simulink model "atrias_HW_boom_nmSt_kinSw_v3"  (R2015a)
settings: Solver=ode4  StartTime=0.0  StopTime=inf  FixedStep=sample_time  RelTol=1e-3
values from neighbouring files (symbols this model uses):
  control_start_time = 15    [setParams.m]
  flag_CtrlMode = 0    [setParams.m]
  kinSw_alpha_start = 130*pi/180    (= 2.26892802759)    [setParams.m]
  kinSw_alpha_tgt = 70*pi/180    (= 1.2217304764)    [setParams.m]
  kinSw_t_start = 0.5    [setParams.m]
  poser_LLegAlp = (initial_l_leg_angle -pi/2)*180/pi    (= 105)    [setParams.m]
  poser_LLegLen = initial_l_leg_length    (= 0.8)    [setParams.m]
  poser_RLegAlp = (initial_r_leg_angle -pi/2)*180/pi    (= 75)    [setParams.m]
  poser_RLegLen = initial_r_leg_length    (= 0.8)    [setParams.m]
  tune_kinSw_alpha_start = kinSw_alpha_start*180/pi    (= 130)    [setParams.m]
  tune_kinSw_alpha_tgt = kinSw_alpha_tgt*180/pi    (= 70)    [setParams.m]
  tune_kinSw_len_min = kinSw_len_min    (= 0.6)    [setParams.m]
  tune_kinSw_len_tgt = kinSw_len_tgt    (= 0.9)    [setParams.m]
  tune_M1_G = 9.5    [setParams.m]
  tune_M3_0 = CtrlPar_theta0*180/pi    [setParams.m]
  tune_M3_D = St_GainDTh_HFL*5    [setParams.m]
  tune_M3_P = St_GainTh_HFL*5    [setParams.m]
  tune_M4_G = 1    [setParams.m]
undefined symbols (not defined in the file or in its folder): A1_notch_f1, A2_notch_f1, A_kalman_fourbar_gear, A_lpf_dtau, B1_lpf_dtau, B1_notch_f1, B2_lpf_dtau, B2_notch_f1, B_kalman_fourbar_gear, boom_mount_angle, boom_mount_to_center_diagonal, c_jointstop, C_kalman_fourbar_gear, contactThr, d_vertical_com, delta_phi_max, delta_phi_max_buffer, delta_phi_max_dropoff, delta_phi_min, Discrete, FmaxBFSH, FmaxGLU, FmaxHAM, FmaxHFL, FmaxRF, FmaxVAS, FPCtrlPar, g, gain_nodes_sea_torque, HIP_MTR_MAX_CONT_TORQUE, initial_dx_estimate, j_motor, k_leg_spring, K_notch_f1, k_sea, kalman_load_to_deflect_transmission, kd_lateral, kd_motor, kd_shin_max, kd_shin_min, kd_splay_max, kd_splay_min, kd_thigh_max, kd_thigh_min, kp_lateral, kp_motor, kp_sea_torque, kp_shin_max, kp_shin_min, kp_splay_max, kp_splay_min, kp_thigh_max, kp_thigh_min, l_boom, l_seg, l_v, lateral_motor_efficiency, lateral_offset, lateral_target_angle_right, lateral_transition_force ... (+123)
libraries: simulink_extras x28, simulink x11, ctrlSharedLib x4
(part 3 of 8)

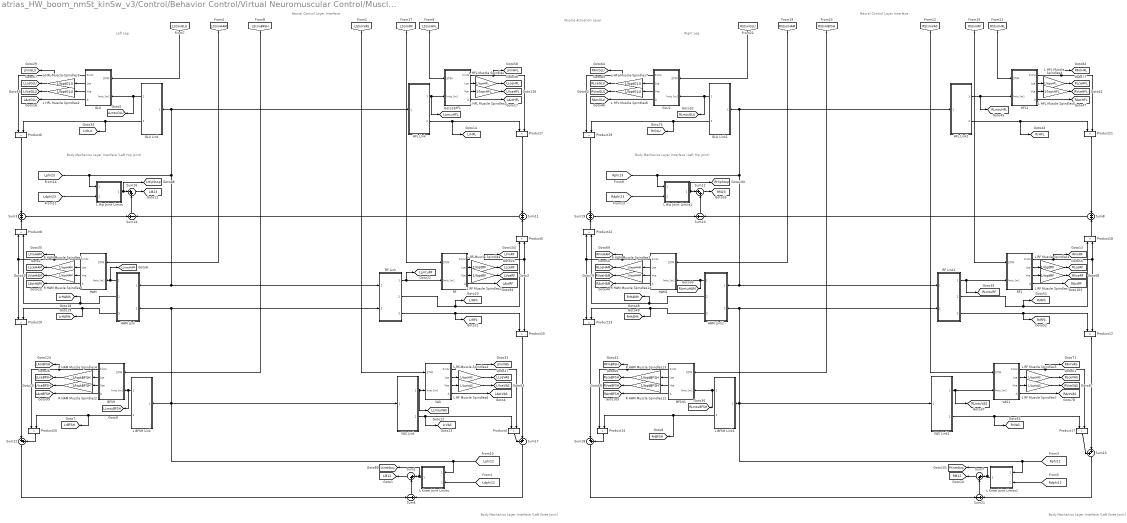
== system atrias_HW_boom_nmSt_kinSw_v3/Control/Behavior Control/Virtual Neuromuscular Control/Muscle Layer ==
  note: Left Leg
  note: Neural Control Layer Interface
  note: Muscle Actuation Layer
  note: Body Mechanics Layer
      | Interface (Left Hip Joint)
  note: Body Mechanics Layer
      | Interface (Left Knee Joint)
  note: Right Leg
  note: Neural Control Layer Interface
  note: Body Mechanics Layer
      | Interface (Left Hip Joint)
  note: Body Mechanics Layer
      | Interface (Left Knee Joint)
  BFSH : Subsystem
  BFSH1 : Subsystem
  GLU : Subsystem
  GLU Link : Subsystem
  GLU Link1 : Subsystem
  GLU1 : Subsystem
  HAM : Subsystem
  HAM Link : Subsystem
  HAM Link1 : Subsystem
  HAM1 : Subsystem
  HFL : Subsystem
  HFL Link : Subsystem
  HFL Link1 : Subsystem
  HFL1 : Subsystem
  L BFSH Link : Subsystem
  L BFSH Link1 : Subsystem
  L HFL Muscle Spindles{,1,4..5} (4 alike) : Gain  Gain=1/loptHFL
  L HFL Muscle Spindles{2..3,6..7} (4 alike) : Gain  Gain=1/loptGLU
  L Hip Joint Limits : Subsystem
  L Hip Joint Limits1 : Subsystem
  L Knee Joint Limits : Subsystem
  L Knee Joint Limits1 : Subsystem
  L RF Muscle Spindles{,1..3} (4 alike) : Gain  Gain=1/loptRF
  L RF Muscle Spindles{4..7} (4 alike) : Gain  Gain=1/loptVAS
  Product{4..9,12,14..15,17..23} (16 alike) : Product  RndMeth=Zero
  R HAM Muscle Spindles{1,3,6,14} (4 alike) : Gain  Gain=1/loptHAM
  R HAM Muscle Spindles{2,4,12..13} (4 alike) : Gain  Gain=1/loptBFSH
  RF : Subsystem
  RF Link : Subsystem
  RF Link1 : Subsystem
  RF1 : Subsystem
  Sum{1,7,12,16,18,22} (6 alike) : Sum  Inputs=|++
  Sum10 : Sum  Inputs=+-
  Sum{3,8,11,19} (4 alike) : Sum
  Sum13 : Sum  Inputs=++|
  Sum14 : Sum  Inputs=+-
  Sum17 : Sum  Inputs=++|
  Sum21 : Sum  Inputs=-+
  Sum5 : Sum  Inputs=-+
  VAS : Subsystem
  VAS Link : Subsystem
  VAS Link1 : Subsystem
  VAS1 : Subsystem
  tag scope: LActBFSH=global, LActGLU=global, LActHAM=global, LActHFL=global, LActRF=global, LActVAS=global, LFmBFSH=global, LFmGLU=global, LFmHAM=global, LFmHFL=global, LFmRF=global, LFmVAS=global, LHipStop=global, LKneeStop=global, LLceBFSH=global, LLceGLU=global, LLceHAM=global, LLceHFL=global, LLceRF=global, LLceVAS=global, LLmtuBFSH=global, LLmtuGLU=global, LLmtuHAM=global, LLmtuHFL=global, LLmtuRF=global, LLmtuVAS=global, LM12=global, LM23=global, LVceBFSH=global, LVceGLU=global, LVceHAM=global, LVceHFL=global, LVceRF=global, LVceVAS=global, LrBFSH=global, LrGLU=global, LrHAMh=global, LrHAMk=global, LrHFL=global, LrRFh=global, LrRFk=global, LrVAS=global, RActBFSH=global, RActGLU=global, RActHAM=global, RActHFL=global, RActRF=global, RActVAS=global, RFmBFSH=global, RFmGLU=global, RFmHAM=global, RFmHFL=global, RFmRF=global, RFmVAS=global, RHipStop=global, RKneeStop=global, RLceBFSH=global, RLceGLU=global, RLceHAM=global, RLceHFL=global, RLceRF=global, RLceVAS=global, RLmtuBFSH=global, RLmtuGLU=global, RLmtuHAM=global, RLmtuHFL=global, RLmtuRF=global, RLmtuVAS=global, RM12=global, RM23=global, RVceBFSH=global, RVceGLU=global, RVceHAM=global, RVceHFL=global, RVceRF=global, RVceVAS=global, RrBFSH=global, RrGLU=global, RrHAMh=global, RrHAMk=global, RrHFL=global, RrRFh=global, RrRFk=global, RrVAS=global
  wires:
  [Lphi12] -> L Knee Joint Limits/1(phi [rad]1), VAS Link/1(phi23 [rad]), RF Link/2(phi23 [rad]), HAM Link/2(phi23 [rad]), L BFSH Link/1(phi23 [rad])
  [LStimHAM] -> HAM/1(STIM)
  HAM/1(Fmtc) -> Product9/1, Product8/1, [LFmHAM]
  HAM/2(Lce) -> R HAM Muscle Spindles1/1
  HFL/1(Fmtc) -> Product7/2, [LFmHFL]
  HFL/2(Lce) -> L HFL Muscle Spindles/1
  [LStimHFL] -> HFL/1(STIM)
  GLU/1(Fmtc) -> Product6/1, [LFmGLU]
  [LStimGLU] -> GLU/1(STIM)
  Sum16/1 -> [LM23]
  [Ldphi12] -> L Knee Joint Limits/2(dphi [rad/s]1)
  VAS Link/1(lmtu [m]) -> VAS/2(lmtc [m]), [LLmtuVAS]
  HAM Link/1(lmtu [m]) -> HAM/2(lmtc [m]), [LLmtuHAM]
  HAM Link/2(lever34 [m]) -> Product8/2, [LrHAMh]
  HAM Link/3(lever23 [m]) -> Product9/2, [LrHAMk]
  Sum3/1 -> Sum14/1
  [Lphi23] -> L Hip Joint Limits/1(phi [rad]1), HFL Link/1(phi34 [rad]), GLU Link/1(phi34 [rad]), RF Link/1(phi34 [rad]), HAM Link/1(phi34 [rad])
  VAS/4(A) -> [LActVAS]
  VAS/1(Fmtc) -> Product4/2, [LFmVAS]
  Sum1/1 -> [LM12]
  L Knee Joint Limits/1(M_stop [Nm]1) -> Sum1/1, [LKneeStop]
  Sum5/1 -> Sum1/2
  VAS Link/2(lever [m]) -> [LrVAS], Product4/1
  Sum22/1 -> Sum5/1
  HAM/4(A) -> [LActHAM]
  Product8/1 -> Sum3/2
  Product6/1 -> Sum3/1
  GLU Link/1(lmtu [m]) -> GLU/2(lmtc [m]), [LLmtuGLU]
  GLU Link/2(lever [m]) -> Product6/2, [LrGLU]
  GLU/4(A) -> [LActGLU]
  [Ldphi23] -> L Hip Joint Limits/2(dphi [rad/s]1)
  L Hip Joint Limits/1(M_stop [Nm]1) -> [LHipStop], Sum16/1
  Sum14/1 -> Sum16/2
  HFL Link/1(lmtu [m]) -> HFL/2(lmtc [m]), [LLmtuHFL]
  HFL/4(A) -> [LActHFL]
  HFL Link/2(lever [m]) -> Product7/1, [LrHFL]
  [LStimVAS] -> VAS/1(STIM)
  GLU/2(Lce) -> L HFL Muscle Spindles3/1
  GLU/3(Vce) -> L HFL Muscle Spindles2/1
  HAM/3(Vce) -> R HAM Muscle Spindles6/1
  VAS/3(Vce) -> L RF Muscle Spindles6/1
  VAS/2(Lce) -> L RF Muscle Spindles4/1
  HFL/3(Vce) -> L HFL Muscle Spindles1/1
  RF/4(A) -> [LActRF]
  RF/3(Vce) -> L RF Muscle Spindles2/1
  RF/2(Lce) -> L RF Muscle Spindles/1
  RF Link/1(lmtu [m]) -> [LLmtuRF], RF/2(lmtc [m])
  RF Link/2(lever34 [m]) -> Product5/1, [LrRFh]
  RF Link/3(lever23 [m]) -> Product15/1, [LrRFk]
  [LStimRF] -> RF/1(STIM)
  Product7/1 -> Sum11/1
  Product5/1 -> Sum11/2
  Product15/1 -> Sum17/2
  Sum17/1 -> Sum5/2
  Product4/1 -> Sum17/1
  [LStimBFSH] -> BFSH/1(STIM)
  L BFSH Link/1(lmtu [m]) -> BFSH/2(lmtc [m]), [LLmtuBFSH]
  L BFSH Link/2(lever [m]) -> [LrBFSH], Product20/2
  BFSH/4(A) -> [LActBFSH]
  BFSH/2(Lce) -> R HAM Muscle Spindles4/1
  BFSH/3(Vce) -> R HAM Muscle Spindles2/1
  Product20/1 -> Sum22/2
  Product9/1 -> Sum22/1
  L HFL Muscle Spindles1/1 -> [LVceHFL]
  L HFL Muscle Spindles2/1 -> [LVceGLU]
  L HFL Muscle Spindles3/1 -> [LLceGLU]
  L RF Muscle Spindles6/1 -> [LVceVAS]
  RF/1(Fmtc) -> Product5/2, Product15/2, [LFmRF]
  BFSH/1(Fmtc) -> Product20/1, [LFmBFSH]
  L HFL Muscle Spindles/1 -> [LLceHFL]
  R HAM Muscle Spindles1/1 -> [LLceHAM]
  R HAM Muscle Spindles6/1 -> [LVceHAM]
  L RF Muscle Spindles/1 -> [LLceRF]
  L RF Muscle Spindles2/1 -> [LVceRF]
  R HAM Muscle Spindles4/1 -> [LLceBFSH]
  R HAM Muscle Spindles2/1 -> [LVceBFSH]
  L RF Muscle Spindles4/1 -> [LLceVAS]
  [Rphi12] -> L Knee Joint Limits1/1(phi [rad]1), VAS Link1/1(phi23 [rad]), HAM Link1/2(phi23 [rad]), RF Link1/2(phi23 [rad]), L BFSH Link1/1(phi23 [rad])
  [RStimHAM] -> HAM1/1(STIM)
  HAM1/1(Fmtc) -> Product23/1, Product22/1, [RFmHAM]
  HAM1/2(Lce) -> R HAM Muscle Spindles3/1
  HFL1/1(Fmtc) -> Product21/2, [RFmHFL]
  HFL1/2(Lce) -> L HFL Muscle Spindles4/1
  [RStimHFL] -> HFL1/1(STIM)
  GLU1/1(Fmtc) -> Product19/1, [RFmGLU]
  [RStimGLU] -> GLU1/1(STIM)
  Sum12/1 -> [RM23]
  [Rdphi12] -> L Knee Joint Limits1/2(dphi [rad/s]1)
  VAS Link1/1(lmtu [m]) -> VAS1/2(lmtc [m]), [RLmtuVAS]
  HAM Link1/1(lmtu [m]) -> HAM1/2(lmtc [m]), [RLmtuHAM]
  HAM Link1/2(lever34 [m]) -> Product22/2, [RrHAMh]
  HAM Link1/3(lever23 [m]) -> Product23/2, [RrHAMk]
  Sum19/1 -> Sum10/1
  [Rphi23] -> L Hip Joint Limits1/1(phi [rad]1), HFL Link1/1(phi34 [rad]), GLU Link1/1(phi34 [rad]), RF Link1/1(phi34 [rad]), HAM Link1/1(phi34 [rad])
  VAS1/4(A) -> [RActVAS]
  VAS1/1(Fmtc) -> Product17/2, [RFmVAS]
  Sum7/1 -> [RM12]
  L Knee Joint Limits1/1(M_stop [Nm]1) -> Sum7/1, [RKneeStop]
  Sum21/1 -> Sum7/2
  VAS Link1/2(lever [m]) -> [RrVAS], Product17/1
  Sum18/1 -> Sum21/1
  HAM1/4(A) -> [RActHAM]
  Product22/1 -> Sum19/2
  Product19/1 -> Sum19/1
  GLU Link1/1(lmtu [m]) -> GLU1/2(lmtc [m]), [RLmtuGLU]
  GLU Link1/2(lever [m]) -> Product19/2, [RrGLU]
  GLU1/4(A) -> [RActGLU]
  [Rdphi23] -> L Hip Joint Limits1/2(dphi [rad/s]1)
  L Hip Joint Limits1/1(M_stop [Nm]1) -> [RHipStop], Sum12/1
  Sum10/1 -> Sum12/2
  HFL Link1/1(lmtu [m]) -> [RLmtuHFL], HFL1/2(lmtc [m])
  HFL1/4(A) -> [RActHFL]
  HFL Link1/2(lever [m]) -> Product21/1, [RrHFL]
  [RStimVAS] -> VAS1/1(STIM)
  GLU1/2(Lce) -> L HFL Muscle Spindles7/1
  GLU1/3(Vce) -> L HFL Muscle Spindles6/1
  HAM1/3(Vce) -> R HAM Muscle Spindles14/1
  VAS1/3(Vce) -> L RF Muscle Spindles7/1
  VAS1/2(Lce) -> L RF Muscle Spindles5/1
  HFL1/3(Vce) -> L HFL Muscle Spindles5/1
  RF1/4(A) -> [RActRF]
  RF1/3(Vce) -> L RF Muscle Spindles3/1
  RF1/2(Lce) -> L RF Muscle Spindles1/1
  RF Link1/1(lmtu [m]) -> RF1/2(lmtc [m]), [RLmtuRF]
  RF Link1/2(lever34 [m]) -> Product18/1, [RrRFh]
  RF Link1/3(lever23 [m]) -> [RrRFk], Product12/1
  [RStimRF] -> RF1/1(STIM)
  Sum8/1 -> Sum10/2
  Product21/1 -> Sum8/1
  Product18/1 -> Sum8/2
  Product12/1 -> Sum13/2
  Sum13/1 -> Sum21/2
  Product17/1 -> Sum13/1
  [RStimBFSH] -> BFSH1/1(STIM)
  L BFSH Link1/1(lmtu [m]) -> BFSH1/2(lmtc [m]), [RLmtuBFSH]
  L BFSH Link1/2(lever [m]) -> [RrBFSH], Product14/2
  BFSH1/4(A) -> [RActBFSH]
  BFSH1/2(Lce) -> R HAM Muscle Spindles13/1
  BFSH1/3(Vce) -> R HAM Muscle Spindles12/1
  Product14/1 -> Sum18/2
  Product23/1 -> Sum18/1
  L HFL Muscle Spindles5/1 -> [RVceHFL]
  L HFL Muscle Spindles6/1 -> [RVceGLU]
  L HFL Muscle Spindles7/1 -> [RLceGLU]
  L RF Muscle Spindles7/1 -> [RVceVAS]
  RF1/1(Fmtc) -> Product18/2, Product12/2, [RFmRF]
  BFSH1/1(Fmtc) -> Product14/1, [RFmBFSH]
  L HFL Muscle Spindles4/1 -> [RLceHFL]
  R HAM Muscle Spindles3/1 -> [RLceHAM]
  R HAM Muscle Spindles14/1 -> [RVceHAM]
  L RF Muscle Spindles1/1 -> [RLceRF]
  L RF Muscle Spindles3/1 -> [RVceRF]
  R HAM Muscle Spindles13/1 -> [RLceBFSH]
  R HAM Muscle Spindles12/1 -> [RVceBFSH]
  L RF Muscle Spindles5/1 -> [RLceVAS]
  Sum11/1 -> Sum14/2

== system atrias_HW_boom_nmSt_kinSw_v3/Control/Behavior Control/Virtual Neuromuscular Control/Neural Control Layer ==
  note: Neural Control Layer
      | (Sagittal Plane)
  Constant1 : Constant  Value=zeros(4,1)  OutDataTypeStr=boolean
  Constant18 : Constant  OutDataTypeStr=boolean
  Constant2 : Constant  Value=zeros(4,1)  OutDataTypeStr=boolean
  Constant3 : Constant  OutDataTypeStr=boolean
  Demux1 : Demux  Outputs=6
  Demux3 : Demux  Outputs=6
  L Stance Phase (sagittal) : Subsystem  TreatAsAtomicUnit=on
  "L Stance, Swing, Trans (sagittal)" : Subsystem
  MDelay{1..4} (4 alike) : Delay  DelayLength=MidDelay_discrete  InitialCondition=0  SampleTime=sample_time
  Mux1 : Mux  Inputs=2
  Mux2 : Mux  Inputs=2
  R Stance Phase (sagittal) : Subsystem  TreatAsAtomicUnit=on
  "R Stance, Swing, Trans (sagittal)" : Subsystem
  Saturation1 : Saturate  UpperLimit=1  LowerLimit=0.01  ZeroCross=off
  Saturation10 : Saturate  UpperLimit=1  LowerLimit=0.01  ZeroCross=off
  tag scope: LAct=global, LStance=global, LStimBFSH=global, LStimGLU=global, LStimHAM=global, LStimHFL=global, LStimRF=global, LStimVAS=global, LSwingPhase=global, RAct=global, RStance=global, RStimBFSH=global, RStimGLU=global, RStimHAM=global, RStimHFL=global, RStimRF=global, RStimVAS=global, RSwingPhase=global
  wires:
  [StCtrlPar] -> L Stance Phase (sagittal)/1(CtrlPar)
  [LFmVAS] -> MDelay2/1
  MDelay2/1 -> MDelay3/1
  [LLceBFSH] -> L Stance Phase (sagittal)/5(LceBFSH)
  Constant18/1 -> L Stance Phase (sagittal)/Enable, [LStance]
  Saturation10/1 -> Demux3/1
  Demux3/1 -> [LStimHFL]  "HFL"
  Demux3/2 -> [LStimGLU]  "GLU"
  Demux3/3 -> [LStimHAM]  "HAM"
  Demux3/4 -> [LStimRF]  "RF"
  Demux3/5 -> [LStimVAS]  "VAS"
  Demux3/6 -> [LStimBFSH]  "BFSH"
  L Stance Phase (sagittal)/1(S_St_0) -> "L Stance, Swing, Trans (sagittal)"/2(S_0_St)
  L Stance Phase (sagittal)/2(S_M1 [VAS]) -> "L Stance, Swing, Trans (sagittal)"/3(S_M1)
  L Stance Phase (sagittal)/3(S_M2 [VAS BFSH]) -> "L Stance, Swing, Trans (sagittal)"/4(S_M2)
  [theta] -> Mux2/1
  [dtheta] -> Mux2/2
  [theta_tgt] -> L Stance Phase (sagittal)/2(theta_tgt [rad])
  [LLLoad] -> "L Stance, Swing, Trans (sagittal)"/1(ILLoad)
  L Stance Phase (sagittal)/4(S_M3 [HFL GLU HAM]) -> "L Stance, Swing, Trans (sagittal)"/5(S_M3)
  Mux2/1 -> L Stance Phase (sagittal)/3(theta dtheta [rad rad/s])
  "L Stance, Swing, Trans (sagittal)"/2(S_Modules) -> [LAct]
  MDelay3/1 -> L Stance Phase (sagittal)/4(FmVAS)
  Constant1/1 -> [LSwingPhase]
  [StCtrlPar] -> R Stance Phase (sagittal)/1(CtrlPar)
  [RFmVAS] -> MDelay1/1
  MDelay1/1 -> MDelay4/1
  [RLceBFSH] -> R Stance Phase (sagittal)/5(LceBFSH)
  Constant3/1 -> R Stance Phase (sagittal)/Enable, [RStance]
  Saturation1/1 -> Demux1/1
  Demux1/1 -> [RStimHFL]  "HFL"
  Demux1/2 -> [RStimGLU]  "GLU"
  Demux1/3 -> [RStimHAM]  "HAM"
  Demux1/4 -> [RStimRF]  "RF"
  Demux1/5 -> [RStimVAS]  "VAS"
  Demux1/6 -> [RStimBFSH]  "BFSH"
  R Stance Phase (sagittal)/1(S_St_0) -> "R Stance, Swing, Trans (sagittal)"/2(S_0_St)
  R Stance Phase (sagittal)/2(S_M1 [VAS]) -> "R Stance, Swing, Trans (sagittal)"/3(S_M1)
  R Stance Phase (sagittal)/3(S_M2 [VAS BFSH]) -> "R Stance, Swing, Trans (sagittal)"/4(S_M2)
  [theta] -> Mux1/1
  [dtheta] -> Mux1/2
  [theta_tgt] -> R Stance Phase (sagittal)/2(theta_tgt [rad])
  [RLLoad] -> "R Stance, Swing, Trans (sagittal)"/1(ILLoad)
  R Stance Phase (sagittal)/4(S_M3 [HFL GLU HAM]) -> "R Stance, Swing, Trans (sagittal)"/5(S_M3)
  Mux1/1 -> R Stance Phase (sagittal)/3(theta dtheta [rad rad/s])
  "R Stance, Swing, Trans (sagittal)"/2(S_Modules) -> [RAct]
  MDelay4/1 -> R Stance Phase (sagittal)/4(FmVAS)
  Constant2/1 -> [RSwingPhase]
  "L Stance, Swing, Trans (sagittal)"/1(S) -> Saturation10/1
  "R Stance, Swing, Trans (sagittal)"/1(S) -> Saturation1/1

== system atrias_HW_boom_nmSt_kinSw_v3/Control/Behavior Control/Virtual Neuromuscular Control/Torque Distribution ==
  note: J^(-T) [tauB; tauF] = [tauH, tauK]
  note: Map Torques
  note: J^(-T) [tauB; tauF] = [tauH, tauK]
  R tauK_des [Nm] : Inport
  R tauH_des [Nm] : Inport  Port=2
  R Jacobian Constant (k) : Inport  Port=3
  L tauK_des [Nm] : Inport  Port=4
  L tauH_des [Nm] : Inport  Port=5
  L Jacobian Constant (k) : Inport  Port=6
  Demux : Demux
  Demux1 : Demux  Outputs=2
  Demux2 : Demux  Outputs=2
  Mux : Mux
  Mux1 : Mux  Inputs=2
  Mux2 : Mux  Inputs=2
  Switch1 : Switch  Criteria=u2 > Threshold
  Switch2 : Switch  Criteria=u2 > Threshold
  Torque Limiter (outside) 1 : Saturate  UpperLimit=max_sagittal_loaded_torque  LowerLimit=-max_sagittal_loaded_torque
      settings: AttributesFormatString=Hi: %<UpperLimit>\nLo: %<LowerLimit>
  Torque Limiter (outside) 2 : Saturate  UpperLimit=max_sagittal_loaded_torque  LowerLimit=-max_sagittal_loaded_torque
      settings: AttributesFormatString=Hi: %<UpperLimit>\nLo: %<LowerLimit>
  Torque Limiter (outside) 3 : Saturate  UpperLimit=max_sagittal_unloaded_torque  LowerLimit=-max_sagittal_unloaded_torque
      settings: AttributesFormatString=Hi: %<UpperLimit>\nLo: %<LowerLimit>
  Torque Limiter (outside) 4 : Saturate  UpperLimit=max_sagittal_unloaded_torque  LowerLimit=-max_sagittal_unloaded_torque
      settings: AttributesFormatString=Hi: %<UpperLimit>\nLo: %<LowerLimit>
  map_tau_L : MATLAB Function  TreatAsAtomicUnit=on
  map_tau_R : MATLAB Function  TreatAsAtomicUnit=on
  mech limit avoidance1 : Subsystem  Commented=on
  R tauB [Nm] : Outport
  R tauF [Nm] : Outport  Port=2
  R J_inv_transpose [2x2] : Outport  Port=3
  L tauB [Nm] : Outport  Port=4
  L tauF [Nm] : Outport  Port=5
  L J_inv_transpose [2x2] : Outport  Port=6
  wires:
  R Jacobian Constant (k)/1 -> map_tau_R/3(k)
  map_tau_R/3(Jinv_trans) -> R J_inv_transpose [2x2]/1
  L Jacobian Constant (k)/1 -> map_tau_L/3(k)
  map_tau_L/3(Jinv_trans) -> L J_inv_transpose [2x2]/1
  map_tau_L/1(tauB) -> Mux2/1
  map_tau_L/2(tauF) -> Mux2/2
  Mux/1 -> Demux/1
  Demux/1 -> [RtauH]
  R tauH_des [Nm]/1 -> Mux/1
  R tauK_des [Nm]/1 -> Mux/2
  L tauH_des [Nm]/1 -> Mux/3
  L tauK_des [Nm]/1 -> Mux/4
  Demux/2 -> [RtauK]
  Demux/3 -> [LtauH]
  Demux/4 -> [LtauK]
  [RtauH] -> map_tau_R/1(tauH_des)
  [RtauK] -> map_tau_R/2(tauK_des)
  [LtauH] -> map_tau_L/1(tauH_des)
  [LtauK] -> map_tau_L/2(tauK_des)
  Switch1/1 -> Demux1/1
  [LFootCnt] -> Switch1/2
  Mux2/1 -> Torque Limiter (outside) 1/1, Torque Limiter (outside) 3/1
  Torque Limiter (outside) 3/1 -> Switch1/3
  Torque Limiter (outside) 1/1 -> Switch1/1
  Demux1/2 -> L tauF [Nm]/1
  Demux1/1 -> L tauB [Nm]/1
  map_tau_R/1(tauB) -> Mux1/1
  map_tau_R/2(tauF) -> Mux1/2
  Switch2/1 -> Demux2/1
  [RFootCnt] -> Switch2/2
  Mux1/1 -> Torque Limiter (outside) 2/1, Torque Limiter (outside) 4/1
  Torque Limiter (outside) 4/1 -> Switch2/3
  Torque Limiter (outside) 2/1 -> Switch2/1
  Demux2/2 -> R tauF [Nm]/1
  Demux2/1 -> R tauB [Nm]/1

== system atrias_HW_boom_nmSt_kinSw_v3/Control/Behavior Control/command routing/(M4) Swing Leg Complensation ==
  RTorques : Inport
  LTorques : Inport  Port=2
  RLeg in Sw [1/0] : Inport  Port=3
  LLeg in Sw [1/0] : Inport  Port=4
  M4_G : Inport  Port=5
  Demux1 : Demux  Outputs=2
  Logical Operator : Logic  Operator=OR  AllPortsSameDT=off  OutDataTypeStr=boolean
  Logical Operator1 : Logic  Operator=NOT  AllPortsSameDT=off  OutDataTypeStr=boolean
  Logical Operator2 : Logic  Operator=NOT  AllPortsSameDT=off  OutDataTypeStr=boolean
  Mux1 : Mux  Inputs=2
  Mux2 : Mux  Inputs=2
  Swing Leg Compensation : Subsystem
  Switch{,1..4} (5 alike) : Switch  Criteria=u2 ~= 0
  RTorques_comp : Outport
  LTorques_comp : Outport  Port=2
  wires:
  [LLegInSw] -> Logical Operator1/1, Switch1/2, Logical Operator/2
  [RLegInSw] -> Logical Operator/1
  Logical Operator/1 -> Switch/2
  [LTorques] -> Mux1/2, Switch2/3, Switch1/3
  [RTorques] -> Switch2/1, Switch1/1, Mux1/1
  Switch1/1 -> Swing Leg Compensation/1(StTorques)
  Logical Operator1/1 -> Switch2/2
  Switch2/1 -> Swing Leg Compensation/2(SwTorques)
  Swing Leg Compensation/1(StTorques_comp) -> Switch4/1, Switch3/1  "St"
  Swing Leg Compensation/2(SwTorques_comp) -> Switch3/3, Switch4/3  "Sw"
  RTorques/1 -> [RTorques]
  LTorques/1 -> [LTorques]
  RLeg in Sw [1/0]/1 -> [RLegInSw]
  LLeg in Sw [1/0]/1 -> [LLegInSw]
  [LLegInSw] -> Logical Operator2/1, Switch3/2
  Logical Operator2/1 -> Switch4/2
  Switch3/1 -> Mux2/1
  Switch4/1 -> Mux2/2
  Mux2/1 -> Switch/1
  Mux1/1 -> Switch/3
  Switch/1 -> Demux1/1
  Demux1/1 -> RTorques_comp/1
  Demux1/2 -> LTorques_comp/1
  M4_G/1 -> [M4_G]
  [M4_G] -> Swing Leg Compensation/3(M4_G)

== system atrias_HW_boom_nmSt_kinSw_v3/Control/Behavior Control/command routing/Desired Torque Derivative (left) ==
  x : Inport
  flight [1/0] : Inport  Port=2
  Detect Change : simulink/Logic and Bit Operations/Detect Change  vinit=0  InputProcessing=Inherited  OutDataTypeStr=boolean
  Gain1 : Gain  Gain=1/sample_time
  Logical Operator : Logic  Operator=NOT  AllPortsSameDT=off  OutDataTypeStr=boolean
  Product : Product
  difference : simulink/Discrete/Difference  ICPrevInput=0.0  InputProcessing=Inherited  OutMin=[]  OutMax=[]  OutDataType=fixdt(1, 16)  OutScaling=2^-10  DoSatur=off
  two_pole_filter : DiscreteTransferFcn  Numerator=[A_lpf_dtau 0 0]  Denominator=[1 B1_lpf_dtau B2_lpf_dtau]  ExternalReset=Either  SampleTime=sample_time
      settings: InputPortMap=u0,r7
  dx/dt : Outport
  wires:
  Logical Operator/1 -> Product/2
  Detect Change/1 -> Logical Operator/1
  Product/1 -> two_pole_filter/1
  difference/1 -> Product/1
  flight [1/0]/1 -> Detect Change/1, two_pole_filter/2
  two_pole_filter/1 -> dx/dt/1
  x/1 -> Gain1/1
  Gain1/1 -> difference/1

== system atrias_HW_boom_nmSt_kinSw_v3/Control/Behavior Control/command routing/Desired Torque Derivative (right) ==
  x : Inport
  flight [1/0] : Inport  Port=2
  Detect Change : simulink/Logic and Bit Operations/Detect Change  vinit=0  InputProcessing=Inherited  OutDataTypeStr=boolean
  Gain1 : Gain  Gain=1/sample_time
  Logical Operator : Logic  Operator=NOT  AllPortsSameDT=off  OutDataTypeStr=boolean
  Product : Product
  difference : simulink/Discrete/Difference  ICPrevInput=0.0  InputProcessing=Inherited  OutMin=[]  OutMax=[]  OutDataType=fixdt(1, 16)  OutScaling=2^-10  DoSatur=off
  two_pole_filter : DiscreteTransferFcn  Numerator=[A_lpf_dtau 0 0]  Denominator=[1 B1_lpf_dtau B2_lpf_dtau]  ExternalReset=Either  SampleTime=sample_time
      settings: InputPortMap=u0,r7
  dx/dt : Outport
  wires:
  Logical Operator/1 -> Product/2
  Detect Change/1 -> Logical Operator/1
  Product/1 -> two_pole_filter/1
  difference/1 -> Product/1
  flight [1/0]/1 -> Detect Change/1, two_pole_filter/2
  two_pole_filter/1 -> dx/dt/1
  x/1 -> Gain1/1
  Gain1/1 -> difference/1

== system atrias_HW_boom_nmSt_kinSw_v3/Control/Behavior Control/kinematic swing leg controller/Back//Front Motor PD ==
  Desired Position [rad] [back front] : Inport
  Desired Velocity [rad/s] [back front] : Inport  Port=2
  Desired Acceleration [rad/s^2] [back front] : Inport  Port=3
  Measured Position [rad] [back front] : Inport  Port=4
  Measured Velocity [rad/s] [back front] : Inport  Port=5
  Right/Left Leg [1/0] : Inport  Port=6
  Friction Compensation : Subsystem
  Product : Product
  Sum1 : Sum  Inputs=|++
  Sum2 : Sum  Inputs=|++
  Sum7 : Sum  Inputs=|+-
  Sum8 : Sum  Inputs=|+-
  Sum9 : Sum
  kd : Gain  Gain=kd_motor
  kp : Gain  Gain=kp_motor
  reflected inertia : Constant  Value=j_motor
  Commanded Torque [Nm] [back front] : Outport
  wires:
  kp/1 -> Sum9/1
  Sum7/1 -> kp/1
  Measured Position [rad] [back front]/1 -> Sum7/2
  Sum9/1 -> Sum1/1
  Sum8/1 -> kd/1
  Desired Position [rad] [back front]/1 -> Sum7/1
  kd/1 -> Sum9/2
  Measured Velocity [rad/s] [back front]/1 -> Sum8/2
  Sum1/1 -> Sum2/1
  Desired Acceleration [rad/s^2] [back front]/1 -> Product/1
  Product/1 -> Sum1/2
  Right/Left Leg [1/0]/1 -> Friction Compensation/1(Right/Left [1/0])
  Sum2/1 -> Commanded Torque [Nm] [back front]/1
  Desired Velocity [rad/s] [back front]/1 -> Friction Compensation/2(Commanded Velocity [rad/s] [back front]), Sum8/1
  reflected inertia/1 -> Product/2
  Friction Compensation/1(Friction Compensation [Nm]) -> Sum2/2

== system atrias_HW_boom_nmSt_kinSw_v3/Control/Behavior Control/kinematic swing leg controller/Desired Torque Derivative (right) ==
  x : Inport
  flight [1/0] : Inport  Port=2
  Detect Change : simulink/Logic and Bit Operations/Detect Change  vinit=0  InputProcessing=Inherited  OutDataTypeStr=boolean
  Gain1 : Gain  Gain=1/sample_time
  Logical Operator : Logic  Operator=NOT  AllPortsSameDT=off  OutDataTypeStr=boolean
  Product : Product
  difference : simulink/Discrete/Difference  ICPrevInput=0.0  InputProcessing=Inherited  OutMin=[]  OutMax=[]  OutDataType=fixdt(1, 16)  OutScaling=2^-10  DoSatur=off
  two_pole_filter : DiscreteTransferFcn  Numerator=[A_lpf_dtau 0 0]  Denominator=[1 B1_lpf_dtau B2_lpf_dtau]  ExternalReset=Either  SampleTime=sample_time
      settings: InputPortMap=u0,r7
  two_pole_filter1 : DiscreteTransferFcn  Numerator=[A_lpf_dtau 0 0]  Denominator=[1 B1_lpf_dtau B2_lpf_dtau]  ExternalReset=Either  SampleTime=sample_time
      settings: InputPortMap=u0,r7
  dx/dt : Outport
  ddx/ddt : Outport  Port=2
  wires:
  Logical Operator/1 -> Product/2
  Detect Change/1 -> Logical Operator/1
  Product/1 -> two_pole_filter/1
  difference/1 -> Product/1
  flight [1/0]/1 -> two_pole_filter1/2, two_pole_filter/2, Detect Change/1
  two_pole_filter/1 -> two_pole_filter1/1, dx/dt/1
  x/1 -> Gain1/1
  Gain1/1 -> difference/1
  two_pole_filter1/1 -> ddx/ddt/1

== system atrias_HW_boom_nmSt_kinSw_v3/Control/Behavior Control/kinematic swing leg controller/Enabled Subsystem1 ==
  In1 : Inport
  In2 : Inport  Port=2
  Enable : EnablePort
  Out1 : Outport  InitialOutput=0
  Out2 : Outport  Port=2  InitialOutput=0
  wires:
  In1/1 -> Out1/1
  In2/1 -> Out2/1

== system atrias_HW_boom_nmSt_kinSw_v3/Control/Behavior Control/kinematic swing leg controller/hold ==
  data : Inport
  Trigger : TriggerPort  PortDimensions=1
  Constant : Constant
  SwCtrlOn : Outport  InitialOutput=0
  data_SwStart : Outport  Port=2
  wires:
  data/1 -> data_SwStart/1
  Constant/1 -> SwCtrlOn/1

== system atrias_HW_boom_nmSt_kinSw_v3/Control/Behavior Control/kinematic swing leg controller/swing leg selector ==
  note: swing leg selector
  Ctrl On [1/0] : Inport
  Rstance : Inport  Port=2
  Lstance : Inport  Port=3
  Ralpha : Inport  Port=4
  Lalpha : Inport  Port=5
  Rlength : Inport  Port=6
  Llength : Inport  Port=7
  RBack Gear [rad rad/s] : Inport  Port=8
  RFront Gear [rad rad/s] : Inport  Port=9
  LBack Gear [rad rad/s] : Inport  Port=10
  LFront Gear [rad rad/s] : Inport  Port=11
  alpha_init : Inport  Port=12
  Data Type Conversion : DataTypeConversion
  Data Type Conversion1 : DataTypeConversion
  Data Type Conversion{2..5} (4 alike) : DataTypeConversion  OutDataTypeStr=double
  Demux : Demux  Outputs=7
  Divide1 : Product
  Divide2 : Product
  Divide3 : Product
  LLeg starts DSup : HitCross  HitCrossingOffset=0.5  HitCrossingDirection=rising  ZeroCross=off
  LLeg starts DSup1 : HitCross  HitCrossingOffset=0.5  HitCrossingDirection=rising  ZeroCross=off
  Logical Operator : Logic  AllPortsSameDT=off
  Logical Operator1 : Logic  AllPortsSameDT=off
  Logical Operator2 : Logic  Operator=OR  AllPortsSameDT=off
  Logical Operator3 : Logic  Operator=NOT  AllPortsSameDT=off
  Logical Operator4 : Logic  Operator=NOT  AllPortsSameDT=off
  Logical Operator5 : Logic  Operator=NOT  AllPortsSameDT=off
  Mux1 : Mux  Inputs=5
  Mux2 : Mux  Inputs=2
  Mux3 : Mux  Inputs=2
  Mux4 : Mux  Inputs=5
  Relational Operator : RelationalOperator
  Relational Operator1 : RelationalOperator
  S-R Flip-Flop1 : simulink_extras/Flip Flops/S-R Flip-Flop  initial_condition=0
  Switch1 : Switch  Criteria=u2 ~= 0  OutDataTypeStr=Inherit: Inherit via back propagation  ZeroCross=off
  Switch6 : Switch  Criteria=u2 ~= 0  OutDataTypeStr=Inherit: Inherit via back propagation  ZeroCross=off
  Terminator : Terminator
  start swing [1/0] : Outport
  swing leg (right/left) [1/0] : Outport  Port=2
  flight : Outport  Port=3
  alpha : Outport  Port=4
  length : Outport  Port=5
  Back Gear [rad rad/s] : Outport  Port=6
  Front Gear [rad rad/s] : Outport  Port=7
  alpha_contra : Outport  Port=8
  wires:
  alpha_init/1 -> Relational Operator1/2, Relational Operator/2
  Logical Operator/1 -> Data Type Conversion/1
  [Lalpha] -> Mux1/2, Relational Operator1/1
  Logical Operator1/1 -> Data Type Conversion1/1
  S-R Flip-Flop1/1 -> Logical Operator5/1, Switch6/2, swing leg (right/left) [1/0]/1
  S-R Flip-Flop1/2 -> Terminator/1
  Switch6/1 -> Demux/1
  Rlength/1 -> Mux4/3
  Mux4/1 -> Switch6/1
  Mux1/1 -> Switch6/3
  Llength/1 -> Mux1/3
  Demux/2 -> alpha/1
  Demux/3 -> length/1
  Logical Operator3/1 -> Data Type Conversion4/1
  Logical Operator4/1 -> Data Type Conversion5/1
  RBack Gear [rad rad/s]/1 -> Mux4/4
  RFront Gear [rad rad/s]/1 -> Mux4/5
  LBack Gear [rad rad/s]/1 -> Mux1/4
  LFront Gear [rad rad/s]/1 -> Mux1/5
  Demux/4 -> Mux2/1
  Demux/5 -> Mux2/2
  Demux/6 -> Mux3/1
  Demux/7 -> Mux3/2
  Mux2/1 -> Back Gear [rad rad/s]/1
  Mux3/1 -> Front Gear [rad rad/s]/1
  LLeg starts DSup/1 -> S-R Flip-Flop1/1, Logical Operator2/1
  LLeg starts DSup1/1 -> S-R Flip-Flop1/2, Logical Operator2/2
  Data Type Conversion1/1 -> LLeg starts DSup1/1
  Data Type Conversion/1 -> LLeg starts DSup/1
  [Ralpha] -> Mux4/2, Relational Operator/1
  Lstance/1 -> Data Type Conversion2/1, Logical Operator4/1
  Rstance/1 -> Data Type Conversion3/1, Logical Operator3/1
  Data Type Conversion2/1 -> Logical Operator/2
  Data Type Conversion3/1 -> Logical Operator1/2
  Data Type Conversion4/1 -> Mux4/1
  Data Type Conversion5/1 -> Mux1/1
  Logical Operator2/1 -> start swing [1/0]/1
  Ctrl On [1/0]/1 -> Divide2/1, Divide3/1, Divide1/1
  Demux/1 -> Divide1/2
  Divide1/1 -> flight/1
  Divide2/1 -> Logical Operator/1
  Relational Operator/1 -> Divide2/2
  Divide3/1 -> Logical Operator1/1
  Relational Operator1/1 -> Divide3/2
  Logical Operator5/1 -> Switch1/2
  Ralpha/1 -> [Ralpha]
  Lalpha/1 -> [Lalpha]
  [Ralpha] -> Switch1/1
  [Lalpha] -> Switch1/3
  Switch1/1 -> alpha_contra/1

== system atrias_HW_boom_nmSt_kinSw_v3/Control/Poser/Subsystem/Back//Front Motor PD ==
  Desired Position [rad] [back front] : Inport
  Desired Velocity [rad/s] [back front] : Inport  Port=2
  Desired Acceleration [rad/s^2] [back front] : Inport  Port=3
  Measured Position [rad] [back front] : Inport  Port=4
  Measured Velocity [rad/s] [back front] : Inport  Port=5
  Right/Left Leg [1/0] : Inport  Port=6
  Friction Compensation : Subsystem
  Product : Product
  Sum1 : Sum  Inputs=|++
  Sum2 : Sum  Inputs=|++
  Sum7 : Sum  Inputs=|+-
  Sum8 : Sum  Inputs=|+-
  Sum9 : Sum
  kd : Gain  Gain=kd_motor
  kp : Gain  Gain=kp_motor
  reflected inertia : Constant  Value=j_motor
  Commanded Torque [Nm] [back front] : Outport
  wires:
  kp/1 -> Sum9/1
  Sum7/1 -> kp/1
  Measured Position [rad] [back front]/1 -> Sum7/2
  Sum9/1 -> Sum1/1
  Sum8/1 -> kd/1
  Desired Position [rad] [back front]/1 -> Sum7/1
  kd/1 -> Sum9/2
  Measured Velocity [rad/s] [back front]/1 -> Sum8/2
  Sum1/1 -> Sum2/1
  Desired Acceleration [rad/s^2] [back front]/1 -> Product/1
  Product/1 -> Sum1/2
  Right/Left Leg [1/0]/1 -> Friction Compensation/1(Right/Left [1/0])
  Sum2/1 -> Commanded Torque [Nm] [back front]/1
  Desired Velocity [rad/s] [back front]/1 -> Friction Compensation/2(Commanded Velocity [rad/s] [back front]), Sum8/1
  reflected inertia/1 -> Product/2
  Friction Compensation/1(Friction Compensation [Nm]) -> Sum2/2

== system atrias_HW_boom_nmSt_kinSw_v3/Control/Poser/Subsystem/Back//Front Motor PD1 ==
  Desired Position [rad] [back front] : Inport
  Desired Velocity [rad/s] [back front] : Inport  Port=2
  Desired Acceleration [rad/s^2] [back front] : Inport  Port=3
  Measured Position [rad] [back front] : Inport  Port=4
  Measured Velocity [rad/s] [back front] : Inport  Port=5
  Right/Left Leg [1/0] : Inport  Port=6
  Friction Compensation : Subsystem
  Product : Product
  Sum1 : Sum  Inputs=|++
  Sum2 : Sum  Inputs=|++
  Sum7 : Sum  Inputs=|+-
  Sum8 : Sum  Inputs=|+-
  Sum9 : Sum
  kd : Gain  Gain=kd_motor
  kp : Gain  Gain=kp_motor
  reflected inertia : Constant  Value=j_motor
  Commanded Torque [Nm] [back front] : Outport
  wires:
  kp/1 -> Sum9/1
  Sum7/1 -> kp/1
  Measured Position [rad] [back front]/1 -> Sum7/2
  Sum9/1 -> Sum1/1
  Sum8/1 -> kd/1
  Desired Position [rad] [back front]/1 -> Sum7/1
  kd/1 -> Sum9/2
  Measured Velocity [rad/s] [back front]/1 -> Sum8/2
  Sum1/1 -> Sum2/1
  Desired Acceleration [rad/s^2] [back front]/1 -> Product/1
  Product/1 -> Sum1/2
  Right/Left Leg [1/0]/1 -> Friction Compensation/1(Right/Left [1/0])
  Sum2/1 -> Commanded Torque [Nm] [back front]/1
  Desired Velocity [rad/s] [back front]/1 -> Friction Compensation/2(Commanded Velocity [rad/s] [back front]), Sum8/1
  reflected inertia/1 -> Product/2
  Friction Compensation/1(Friction Compensation [Nm]) -> Sum2/2

== system atrias_HW_boom_nmSt_kinSw_v3/Control/Poser/Subsystem/dtau_des ==
  x : Inport
  Gain1 : Gain  Gain=1/sample_time
  difference : simulink/Discrete/Difference  ICPrevInput=0.0  InputProcessing=Inherited  OutMin=[]  OutMax=[]  OutDataType=fixdt(1, 16)  OutScaling=2^-10  DoSatur=off
  two_pole_filter : DiscreteTransferFcn  Numerator=[A_lpf_dtau 0 0]  Denominator=[1 B1_lpf_dtau B2_lpf_dtau]  SampleTime=sample_time
  dx/dt : Outport
  wires:
  two_pole_filter/1 -> dx/dt/1
  x/1 -> Gain1/1
  difference/1 -> two_pole_filter/1
  Gain1/1 -> difference/1

== system atrias_HW_boom_nmSt_kinSw_v3/Control/Behavior Control/Add Limit Avoidance PD Torques/mechanical limit avoidance/PD Joint Limit ==
  L Scale desired torque : Subsystem
  L mechanical Limit Avoidance Torques (Virtual) : Subsystem
  Mux : Mux
  Mux1 : Mux
  R Mechanical Limit Avoidance Torques (Virtual)1 : Subsystem
  R Scale desired torque : Subsystem
  tau_pd [Nm]x4 : Outport
  des_trq_scale x4 : Outport  Port=2
  tag scope: L_scale_back=global, L_scale_front=global, Ltau_pd_back=global, Ltau_pd_front=global, R_scale_back=global, R_scale_front=global, Rtau_pd_back=global, Rtau_pd_front=global
  wires:
  [Lphi_thigh] -> L mechanical Limit Avoidance Torques (Virtual)/1(phi_thigh [rad])
  [Lphi_shin] -> L mechanical Limit Avoidance Torques (Virtual)/2(phi_shin [rad])
  [Ldphi_thigh] -> L mechanical Limit Avoidance Torques (Virtual)/3(dphi_thigh [rad/s])
  [Ldphi_shin] -> L mechanical Limit Avoidance Torques (Virtual)/4(dphi_shin [rad/s])
  [Rphi_thigh] -> R Mechanical Limit Avoidance Torques (Virtual)1/1(phi_thigh [rad])
  [Rphi_shin] -> R Mechanical Limit Avoidance Torques (Virtual)1/2(phi_shin [rad])
  [Rdphi_thigh] -> R Mechanical Limit Avoidance Torques (Virtual)1/3(dphi_thigh [rad/s])
  [Rdphi_shin] -> R Mechanical Limit Avoidance Torques (Virtual)1/4(dphi_shin [rad/s])
  [Ltau_pd_front] -> Mux/4  "Lthigh"
  [Ltau_pd_back] -> Mux/3  "Lshin"
  [Rtau_pd_front] -> Mux/2  "Rthigh"
  [Rtau_pd_back] -> Mux/1  "Rshin"
  Mux/1 -> tau_pd [Nm]x4/1
  [Rphi_thigh] -> R Scale desired torque/1(phi_thigh [rad])
  [Rphi_shin] -> R Scale desired torque/2(phi_shin [rad])
  [Lphi_thigh] -> L Scale desired torque/1(phi_thigh [rad])
  [Lphi_shin] -> L Scale desired torque/2(phi_shin [rad])
  [L_scale_front] -> Mux1/4
  [L_scale_back] -> Mux1/3
  [R_scale_front] -> Mux1/2
  [R_scale_back] -> Mux1/1
  Mux1/1 -> des_trq_scale x4/1
  R Scale desired torque/1(scale_back) -> [R_scale_back]
  R Scale desired torque/2(scale_front) -> [R_scale_front]
  L Scale desired torque/1(scale_back) -> [L_scale_back]
  L Scale desired torque/2(scale_front) -> [L_scale_front]
  R Mechanical Limit Avoidance Torques (Virtual)1/1(tau_pd_back [Nm]) -> [Rtau_pd_back]
  R Mechanical Limit Avoidance Torques (Virtual)1/2(tau_pd_front [Nm]) -> [Rtau_pd_front]
  L mechanical Limit Avoidance Torques (Virtual)/1(tau_pd_back [Nm]) -> [Ltau_pd_back]
  L mechanical Limit Avoidance Torques (Virtual)/2(tau_pd_front [Nm]) -> [Ltau_pd_front]

== system atrias_HW_boom_nmSt_kinSw_v3/Control/Behavior Control/Virtual Neuromuscular Control/Higher Control Layer/Double Support ==
  LStance : Inport
  RStance : Inport  Port=2
  Lalpha_tgt : Inport  Port=3
  Lphi34 : Inport  Port=4
  Lphi23 : Inport  Port=5
  Ralpha_tgt : Inport  Port=6
  Rphi34 : Inport  Port=7
  Rphi23 : Inport  Port=8
  Abs : Abs  ZeroCross=off
  Abs1 : Abs  ZeroCross=off
  Lalpha' : Fcn  Expr=u(1) - u(2)/2
  Logical Operator1 : Logic  Operator=NOR  AllPortsSameDT=off
  Logical Operator2 : Logic  Operator=NOT  AllPortsSameDT=off
  Logical Operator{3..7} (5 alike) : Logic  AllPortsSameDT=off
  Mux1 : Mux  Inputs=2
  Mux5 : Mux  Inputs=2
  Ralpha' : Fcn  Expr=u(1) - u(2)/2
  Relational Operator : RelationalOperator  Operator=>  ZeroCross=off
  Sum5 : Sum  Inputs=-+|
  Sum7 : Sum  Inputs=-+|
  RonL : Outport
  Flight : Outport  Port=2
  LonR : Outport  Port=3
  DS : Outport  Port=4
  RonL (Flight) : Outport  Port=5
  LonR (Flight) : Outport  Port=6
  wires:
  Lalpha'/1 -> Sum7/2  "Lalpha"
  Mux5/1 -> Lalpha'/1
  Ralpha'/1 -> Sum5/2
  Mux1/1 -> Ralpha'/1
  Sum5/1 -> Abs/1
  Sum7/1 -> Abs1/1
  LStance/1 -> Logical Operator3/1, Logical Operator1/1
  RStance/1 -> Logical Operator3/2, Logical Operator1/2
  Lalpha_tgt/1 -> Sum7/1
  Lphi34/1 -> Mux5/1
  Lphi23/1 -> Mux5/2
  Ralpha_tgt/1 -> Sum5/1
  Rphi34/1 -> Mux1/1
  Rphi23/1 -> Mux1/2
  Logical Operator1/1 -> Flight/1, Logical Operator7/1, Logical Operator6/1
  Abs1/1 -> Relational Operator/1
  Abs/1 -> Relational Operator/2
  Logical Operator4/1 -> RonL/1
  Logical Operator2/1 -> Logical Operator7/2, Logical Operator5/2
  Logical Operator5/1 -> LonR/1
  Relational Operator/1 -> Logical Operator2/1, Logical Operator6/2, Logical Operator4/2
  Logical Operator3/1 -> DS/1, Logical Operator4/1, Logical Operator5/1
  Logical Operator6/1 -> RonL (Flight)/1
  Logical Operator7/1 -> LonR (Flight)/1

== system atrias_HW_boom_nmSt_kinSw_v3/Control/Behavior Control/Virtual Neuromuscular Control/Muscle Layer/BFSH ==
  note: SOLEUS Muscle-Tendon Dynamics
  note: Excitation Contraction Coupling
  STIM : Inport
  lmtc [m] : Inport  Port=2
  1 : Product  Inputs=**  SaturateOnIntegerOverflow=on  InputSameDT=on  OutDataTypeStr=Inherit: Same as first input
  1/lslack : Gain  Gain=1/lslackBFSH  SaturateOnIntegerOverflow=on  OutDataTypeStr=Inherit: Same as input  ParamDataTypeStr=Inherit: Same as input
  BE force-length relation : Subsystem
  CE force-length relation : Subsystem
  CE inverse force-velocity relation : Subsystem
  Constant : Constant  Value=lslackBFSH
  ECC TransferFcn : simulink_extras/Additional Linear/Transfer Fcn (with initial outputs)  N=[1]  D="[mtu_tau  1]"  Y0=mtu_preA  U0=0
      settings: AttributesFormatString=pre-activation: %<Y0>
  Fmax : Gain  Gain=FmaxBFSH  SaturateOnIntegerOverflow=on  OutDataTypeStr=Inherit: Same as input  ParamDataTypeStr=Inherit: Same as input
  Fv = Fse / (A*Fce) : Product  Inputs=*/  SaturateOnIntegerOverflow=on  InputSameDT=on  OutDataTypeStr=Inherit: Same as first input
  Integrator : Integrator  InitialConditionSource=external  LowerSaturationLimit=0.05
  PE force-length relation : Subsystem
  SE force-length relation : Subsystem
  Saturation : Saturate  UpperLimit=1  LowerLimit=0.01
  Sum : Sum  Inputs=|+-  SaturateOnIntegerOverflow=on  InputSameDT=on  OutDataTypeStr=Inherit: Same as first input
  Sum2 : Sum  Inputs=|-+  SaturateOnIntegerOverflow=on  InputSameDT=on  OutDataTypeStr=Inherit: Same as first input
  Sum3 : Sum  SaturateOnIntegerOverflow=on  InputSameDT=on  OutDataTypeStr=Inherit: Same as first input
  Sum4 : Sum  SaturateOnIntegerOverflow=on  InputSameDT=on  OutDataTypeStr=Inherit: Same as first input
  lce/lopt : Gain  Gain=1/loptBFSH  SaturateOnIntegerOverflow=on  OutDataTypeStr=Inherit: Same as input  ParamDataTypeStr=Inherit: Same as input
  vmax*lopt : Gain  Gain=vmaxBFSH*loptBFSH  SaturateOnIntegerOverflow=on  OutDataTypeStr=Inherit: Same as input  ParamDataTypeStr=Inherit: Same as input
  Fmtc : Outport  InitialOutput=0
  Lce : Outport  Port=2  InitialOutput=0
  Vce : Outport  Port=3  InitialOutput=0
  A : Outport  Port=4  InitialOutput=0
  wires:
  Integrator/1 -> Sum/2, lce/lopt/1, Lce/1  "lce"
  Sum/1 -> 1/lslack/1  "lse"
  lce/lopt/1 -> CE force-length relation/1(lce [lopt]), BE force-length relation/1(lce [lopt]), PE force-length relation/1(lce [lopt])
  Fv = Fse / (A*Fce)/1 -> CE inverse force-velocity relation/1(Fv[Fmax])  "fv"
  vmax*lopt/1 -> Integrator/1, Vce/1  "vce"
  lmtc [m]/1 -> Sum2/2, Sum/1  "lmtc"
  Fmax/1 -> Fmtc/1  "Fmtc"
  1/lslack/1 -> SE force-length relation/1(lse [lslack])
  SE force-length relation/1(fse [Fmax]) -> Fmax/1, Sum4/1
  Sum2/1 -> Integrator/2
  Constant/1 -> Sum2/1
  CE force-length relation/1(fce [Fmax]) -> 1/1
  Sum4/1 -> Fv = Fse / (A*Fce)/1
  PE force-length relation/1(fpe [Fmax]) -> Sum3/1
  1/1 -> Sum3/2
  BE force-length relation/1(fbe [Fmax]) -> Sum4/2
  Sum3/1 -> Fv = Fse / (A*Fce)/2
  CE inverse force-velocity relation/1(v[vmax]) -> vmax*lopt/1
  STIM/1 -> ECC TransferFcn/1
  ECC TransferFcn/1 -> Saturation/1
  Saturation/1 -> A/1, 1/2

== system atrias_HW_boom_nmSt_kinSw_v3/Control/Behavior Control/Virtual Neuromuscular Control/Muscle Layer/BFSH1 ==
  note: SOLEUS Muscle-Tendon Dynamics
  note: Excitation Contraction Coupling
  STIM : Inport
  lmtc [m] : Inport  Port=2
  1 : Product  Inputs=**  SaturateOnIntegerOverflow=on  InputSameDT=on  OutDataTypeStr=Inherit: Same as first input
  1/lslack : Gain  Gain=1/lslackBFSH  SaturateOnIntegerOverflow=on  OutDataTypeStr=Inherit: Same as input  ParamDataTypeStr=Inherit: Same as input
  BE force-length relation : Subsystem
  CE force-length relation : Subsystem
  CE inverse force-velocity relation : Subsystem
  Constant : Constant  Value=lslackBFSH
  ECC TransferFcn : simulink_extras/Additional Linear/Transfer Fcn (with initial outputs)  N=[1]  D="[mtu_tau  1]"  Y0=mtu_preA  U0=0
      settings: AttributesFormatString=pre-activation: %<Y0>
  Fmax : Gain  Gain=FmaxBFSH  SaturateOnIntegerOverflow=on  OutDataTypeStr=Inherit: Same as input  ParamDataTypeStr=Inherit: Same as input
  Fv = Fse / (A*Fce) : Product  Inputs=*/  SaturateOnIntegerOverflow=on  InputSameDT=on  OutDataTypeStr=Inherit: Same as first input
  Integrator : Integrator  InitialConditionSource=external  LowerSaturationLimit=0.05
  PE force-length relation : Subsystem
  SE force-length relation : Subsystem
  Saturation : Saturate  UpperLimit=1  LowerLimit=0.01
  Sum : Sum  Inputs=|+-  SaturateOnIntegerOverflow=on  InputSameDT=on  OutDataTypeStr=Inherit: Same as first input
  Sum2 : Sum  Inputs=|-+  SaturateOnIntegerOverflow=on  InputSameDT=on  OutDataTypeStr=Inherit: Same as first input
  Sum3 : Sum  SaturateOnIntegerOverflow=on  InputSameDT=on  OutDataTypeStr=Inherit: Same as first input
  Sum4 : Sum  SaturateOnIntegerOverflow=on  InputSameDT=on  OutDataTypeStr=Inherit: Same as first input
  lce/lopt : Gain  Gain=1/loptBFSH  SaturateOnIntegerOverflow=on  OutDataTypeStr=Inherit: Same as input  ParamDataTypeStr=Inherit: Same as input
  vmax*lopt : Gain  Gain=vmaxBFSH*loptBFSH  SaturateOnIntegerOverflow=on  OutDataTypeStr=Inherit: Same as input  ParamDataTypeStr=Inherit: Same as input
  Fmtc : Outport  InitialOutput=0
  Lce : Outport  Port=2  InitialOutput=0
  Vce : Outport  Port=3  InitialOutput=0
  A : Outport  Port=4  InitialOutput=0
  wires:
  Integrator/1 -> Sum/2, lce/lopt/1, Lce/1  "lce"
  Sum/1 -> 1/lslack/1  "lse"
  lce/lopt/1 -> CE force-length relation/1(lce [lopt]), BE force-length relation/1(lce [lopt]), PE force-length relation/1(lce [lopt])
  Fv = Fse / (A*Fce)/1 -> CE inverse force-velocity relation/1(Fv[Fmax])  "fv"
  vmax*lopt/1 -> Integrator/1, Vce/1  "vce"
  lmtc [m]/1 -> Sum2/2, Sum/1  "lmtc"
  Fmax/1 -> Fmtc/1  "Fmtc"
  1/lslack/1 -> SE force-length relation/1(lse [lslack])
  SE force-length relation/1(fse [Fmax]) -> Fmax/1, Sum4/1
  Sum2/1 -> Integrator/2
  Constant/1 -> Sum2/1
  CE force-length relation/1(fce [Fmax]) -> 1/1
  Sum4/1 -> Fv = Fse / (A*Fce)/1
  PE force-length relation/1(fpe [Fmax]) -> Sum3/1
  1/1 -> Sum3/2
  BE force-length relation/1(fbe [Fmax]) -> Sum4/2
  Sum3/1 -> Fv = Fse / (A*Fce)/2
  CE inverse force-velocity relation/1(v[vmax]) -> vmax*lopt/1
  STIM/1 -> ECC TransferFcn/1
  ECC TransferFcn/1 -> Saturation/1
  Saturation/1 -> A/1, 1/2

== system atrias_HW_boom_nmSt_kinSw_v3/Control/Behavior Control/Virtual Neuromuscular Control/Muscle Layer/GLU ==
  note: SOLEUS Muscle-Tendon Dynamics
  note: Excitation Contraction Coupling
  STIM : Inport
  lmtc [m] : Inport  Port=2
  1 : Product  Inputs=**  SaturateOnIntegerOverflow=on  InputSameDT=on  OutDataTypeStr=Inherit: Same as first input
  1/lslack : Gain  Gain=1/lslackGLU  SaturateOnIntegerOverflow=on  OutDataTypeStr=Inherit: Same as input  ParamDataTypeStr=Inherit: Same as input
  BE force-length relation : Subsystem
  CE force-length relation : Subsystem
  CE inverse force-velocity relation : Subsystem
  Constant : Constant  Value=lslackGLU
  ECC TransferFcn : simulink_extras/Additional Linear/Transfer Fcn (with initial outputs)  N=[1]  D="[mtu_tau  1]"  Y0=mtu_preA  U0=0
      settings: AttributesFormatString=pre-activation: %<Y0>
  Fmax : Gain  Gain=FmaxGLU  SaturateOnIntegerOverflow=on  OutDataTypeStr=Inherit: Same as input  ParamDataTypeStr=Inherit: Same as input
  Fv = Fse / (A*Fce) : Product  Inputs=*/  SaturateOnIntegerOverflow=on  InputSameDT=on  OutDataTypeStr=Inherit: Same as first input
  Integrator : Integrator  InitialConditionSource=external  LowerSaturationLimit=0.05
  PE force-length relation : Subsystem
  SE force-length relation : Subsystem
  Saturation : Saturate  UpperLimit=1  LowerLimit=0.01
  Sum : Sum  Inputs=|+-  SaturateOnIntegerOverflow=on  InputSameDT=on  OutDataTypeStr=Inherit: Same as first input
  Sum2 : Sum  Inputs=|-+  SaturateOnIntegerOverflow=on  InputSameDT=on  OutDataTypeStr=Inherit: Same as first input
  Sum3 : Sum  SaturateOnIntegerOverflow=on  InputSameDT=on  OutDataTypeStr=Inherit: Same as first input
  Sum4 : Sum  SaturateOnIntegerOverflow=on  InputSameDT=on  OutDataTypeStr=Inherit: Same as first input
  lce/lopt : Gain  Gain=1/loptGLU  SaturateOnIntegerOverflow=on  OutDataTypeStr=Inherit: Same as input  ParamDataTypeStr=Inherit: Same as input
  vmax*lopt : Gain  Gain=vmaxGLU*loptGLU  SaturateOnIntegerOverflow=on  OutDataTypeStr=Inherit: Same as input  ParamDataTypeStr=Inherit: Same as input
  Fmtc : Outport  InitialOutput=0
  Lce : Outport  Port=2  InitialOutput=0
  Vce : Outport  Port=3  InitialOutput=0
  A : Outport  Port=4  InitialOutput=0
  wires:
  Integrator/1 -> Sum/2, lce/lopt/1, Lce/1  "lce"
  Sum/1 -> 1/lslack/1  "lse"
  lce/lopt/1 -> CE force-length relation/1(lce [lopt]), BE force-length relation/1(lce [lopt]), PE force-length relation/1(lce [lopt])
  Fv = Fse / (A*Fce)/1 -> CE inverse force-velocity relation/1(Fv[Fmax])  "fv"
  vmax*lopt/1 -> Integrator/1, Vce/1  "vce"
  lmtc [m]/1 -> Sum2/2, Sum/1  "lmtc"
  Fmax/1 -> Fmtc/1  "Fmtc"
  1/lslack/1 -> SE force-length relation/1(lse [lslack])
  SE force-length relation/1(fse [Fmax]) -> Fmax/1, Sum4/1
  Sum2/1 -> Integrator/2
  Constant/1 -> Sum2/1
  CE force-length relation/1(fce [Fmax]) -> 1/1
  Sum4/1 -> Fv = Fse / (A*Fce)/1
  PE force-length relation/1(fpe [Fmax]) -> Sum3/1
  1/1 -> Sum3/2
  BE force-length relation/1(fbe [Fmax]) -> Sum4/2
  Sum3/1 -> Fv = Fse / (A*Fce)/2
  CE inverse force-velocity relation/1(v[vmax]) -> vmax*lopt/1
  STIM/1 -> ECC TransferFcn/1
  ECC TransferFcn/1 -> Saturation/1
  Saturation/1 -> A/1, 1/2

== system atrias_HW_boom_nmSt_kinSw_v3/Control/Behavior Control/Virtual Neuromuscular Control/Muscle Layer/GLU Link ==
  note: GLUTEUS Attachment
  phi34 [rad] : Inport
  Constant : Constant  Value=lslackGLU+loptGLU
  Constant1 : Constant  Value=rGLU
  Constant2 : Constant  Value=phirefGLU
  Gain2 : Gain  Gain=rhoGLU
  Product : Product  RndMeth=Zero
  Sum2 : Sum  Inputs=|+-
  Sum5 : Sum  Inputs=|+-
  lmtu [m] : Outport
  lever [m] : Outport  Port=2
  wires:
  Constant/1 -> Sum5/1
  Sum5/1 -> lmtu [m]/1
  Product/1 -> Gain2/1
  phi34 [rad]/1 -> Sum2/1
  Constant2/1 -> Sum2/2
  Sum2/1 -> Product/1
  Constant1/1 -> Product/2, lever [m]/1
  Gain2/1 -> Sum5/2

== system atrias_HW_boom_nmSt_kinSw_v3/Control/Behavior Control/Virtual Neuromuscular Control/Muscle Layer/GLU Link1 ==
  note: GLUTEUS Attachment
  phi34 [rad] : Inport
  Constant : Constant  Value=lslackGLU+loptGLU
  Constant1 : Constant  Value=rGLU
  Constant2 : Constant  Value=phirefGLU
  Gain2 : Gain  Gain=rhoGLU
  Product : Product  RndMeth=Zero
  Sum2 : Sum  Inputs=|+-
  Sum5 : Sum  Inputs=|+-
  lmtu [m] : Outport
  lever [m] : Outport  Port=2
  wires:
  Constant/1 -> Sum5/1
  Sum5/1 -> lmtu [m]/1
  Product/1 -> Gain2/1
  phi34 [rad]/1 -> Sum2/1
  Constant2/1 -> Sum2/2
  Sum2/1 -> Product/1
  Constant1/1 -> Product/2, lever [m]/1
  Gain2/1 -> Sum5/2
